simulink model "Actividad1_Manipulador_de_un_enlace"  (R2023a)
settings: Solver=VariableStepAuto  StartTime=0.0  StopTime=1000  RelTol=1e-3
settings Model: Creator=alfre  LastModifiedBy=unknown

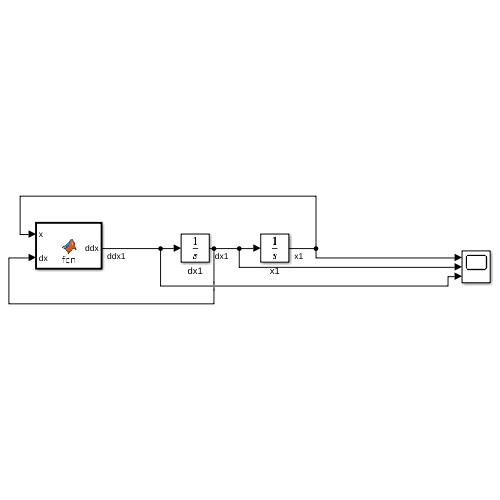
[thumbnail: Simulink's stored preview of the top-level diagram]
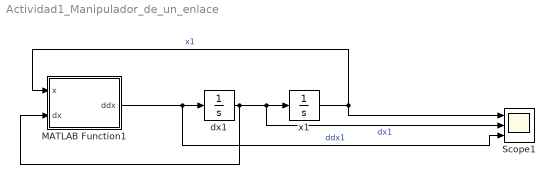
== system Actividad1_Manipulador_de_un_enlace ==
  MATLAB Function1 : MATLAB Function  TreatAsAtomicUnit=on
  Scope1 : Scope  NumInputPorts=3
  dx1 : Integrator  InitialCondition=5  ContinuousStateAttributes="\"dx\""
  x1 : Integrator  ContinuousStateAttributes="\"dx\""
  wires:
  MATLAB Function1/1(ddx) -> Scope1/3, dx1/1  "ddx1"
  dx1/1 -> MATLAB Function1/2(dx), Scope1/2, x1/1  "dx1"
  x1/1 -> MATLAB Function1/1(x), Scope1/1  "x1"

== matlab function Actividad1_Manipulador_de_un_enlace/MATLAB Function1 ==
  data: x input; ddx output; dx input
function ddx = fcn(x, dx)
k = 0.01;
m = 5;
l = 0.36;
g=9.8;
a=l/2;
Tau= 0.0;
J=(4*m*a^2)/3;
ddx= Tau/J- k*dx/J- m*g*a*cos(x)/J;
